simulink model "CANTXmessagesunit"  (R2024a)
settings: Solver=VariableStepAuto  StartTime=0.0  StopTime=10.0  RelTol=1e-3
undefined symbols (not defined in the file or in its folder): canChannel
libraries: canlib x3, canmsglib x2
settings Model: DataDictionary=BMS_System_Arch_dict.sldd  Creator=hirah  LastModifiedBy=hirah

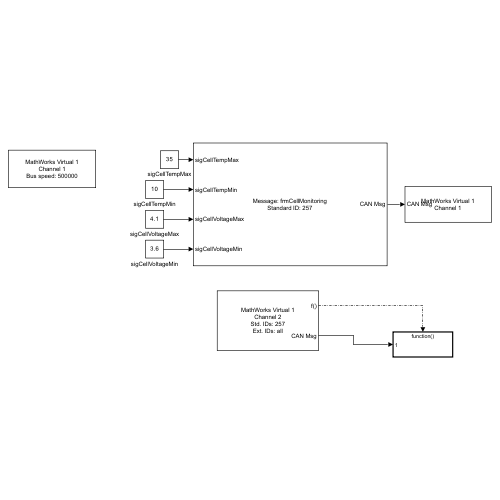
[thumbnail: Simulink's stored preview of the top-level diagram]
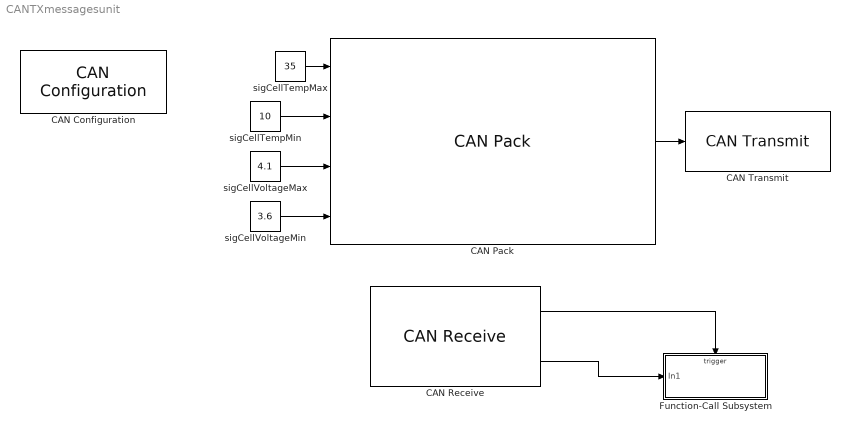
== system CANTXmessagesunit ==
  CAN Configuration : canlib/CAN Configuration  BlockHandle=291.0001  Device=MathWorks Virtual 1 (Channel 1)  DeviceMenu=MathWorks Virtual 1 (Channel 1)  ObjConstructor=canChannel('MathWorks', 'Virtual 1', 1)  BusSpeed=500000  EnableBitParameters=off  AckMode=Normal
  CAN Pack : canmsglib/CAN Pack  CANdbFile=C:\Users\hirah\Downloads\BMS_CAN_Database (5).dbc  MsgList=frmCellMonitoring  MsgName=frmCellMonitoring  MsgIDType=Standard (11-bit identifier)  MsgIdentifier=257  MsgLength=6  Remote=off  ApplyMinMax=off  BusOutput=off  SignalInfo={ 'sigCellTempMax', '32', '8', 'LE', 'unsigned', 'Standard', '0', '1', '-40', '-40', '150'; 'sigCellTempMin', '40', '8', 'LE', 'unsigned', 'Standard', '0', '1', '-40', '-40', '150'; 'sigCellVoltageMax', '0', '16', 'LE', 'unsigned', 'Standard', '0', '0.001', '0', '0', '5'; 'sigCellVoltageMin', '16', '16', 'LE', 'unsigned', 'Standard', '0', '0.001', '0', '0', '5' }
      settings: LibrarySourceBlock=canlib/CAN Pack  DataFormat=manually specified signals
  CAN Receive : canlib/CAN Receive  BlockHandle=298.0001  Device=MathWorks Virtual 1 (Channel 2)  DeviceMenu=MathWorks Virtual 1 (Channel 2)  ObjConstructor=canChannel('MathWorks', 'Virtual 1', 2)  EnableStandardIDsFilter=off  StdIDsCombo=Allow only  StandardIDs=257  EnableExtendedIDsFilter=off  ExtIDsCombo=Allow all  ExtendedIDs=0  SampleTime=0.01  MsgsPerTimestep=all  InternalFilterUpdateStatus=on  BusOutput=off
  CAN Transmit : canlib/CAN Transmit  BlockHandle=301.0001  Device=MathWorks Virtual 1 (Channel 1)  DeviceMenu=MathWorks Virtual 1 (Channel 1)  ObjConstructor=canChannel('MathWorks', 'Virtual 1', 1)  EnableEventTransmit=off  EnablePeriodicTransmit=off  MessagePeriod=1.000
  Function-Call Subsystem : Subsystem  TreatAsAtomicUnit=on
  sigCellTempMax : Constant  Value=35  OutDataTypeStr=int8
  sigCellTempMin : Constant  Value=10  OutDataTypeStr=int8
  sigCellVoltageMax : Constant  Value=4.1  OutDataTypeStr=double
  sigCellVoltageMin : Constant  Value=3.6  OutDataTypeStr=double
  wires:
  sigCellTempMax/1 -> CAN Pack/1
  CAN Pack/1 -> CAN Transmit/1
  sigCellTempMin/1 -> CAN Pack/2
  sigCellVoltageMin/1 -> CAN Pack/4
  CAN Receive/1 -> Function-Call Subsystem/Trigger
  CAN Receive/2 -> Function-Call Subsystem/1(In1)
  sigCellVoltageMax/1 -> CAN Pack/3

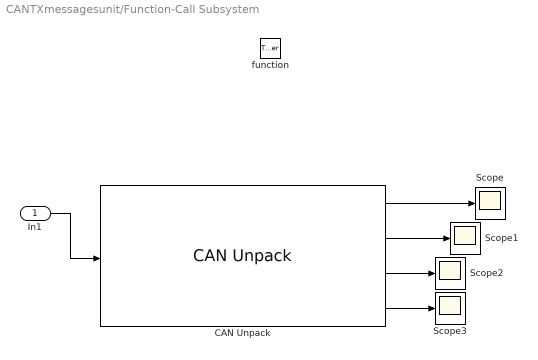
== system CANTXmessagesunit/Function-Call Subsystem ==
  In1 : Inport
  function : TriggerPort  TriggerType=function-call  VariantControl=(inherit)
  CAN Unpack : canmsglib/CAN Unpack  CANdbFile=C:\Users\hirah\Downloads\BMS_CAN_Database (5).dbc  MsgList=frmCellMonitoring  MsgName=frmCellMonitoring  MsgIDType=Standard (11-bit identifier)  MsgIdentifier=257  MsgLength=6  SignalInfo={'sigCellTempMax','32','8','LE','unsigned','Standard','0','1','-40','-40','150';'sigCellTempMin','40','8','LE','unsigned','Standard','0','1','-40','-40','150';'sigCellVoltageMax','0','16','LE','unsigned','Standard','0','0.001','0','0','5';'sigCellVoltageMin','16','16','LE','unsigned','Standard','0','0.001','0','0','5'}  IDPort=off  TimestampPort=off  ErrorPort=off  RemotePort=off  LengthPort=off  StatusPort=off  ApplyMinMax=off
      settings: DataFormat=CANdb specified signals
  Scope{,1..3} (4 alike) : Scope
  wires:
  In1/1 -> CAN Unpack/1
  CAN Unpack/1 -> Scope/1
  CAN Unpack/2 -> Scope1/1
  CAN Unpack/3 -> Scope2/1
  CAN Unpack/4 -> Scope3/1
